simulink model "autosar_swc_actuator"  (R2021a)
settings: Solver=FixedStepDiscrete  StartTime=0.0  StopTime=10.0  FixedStep=0.02  RelTol=1e-3
model workspace (MATLAB code in the model file):
  | HBridgeCmd_LkupTbl = Simulink.LookupTable;
  | HBridgeCmd_LkupTbl.Table.DataType = 'int16';
  | HBridgeCmd_LkupTbl.Table.FieldName = 'Table';
  | HBridgeCmd_LkupTbl.Table.Value = int16( ...
  |   [-2048 -1843 -1638 -1434 -1229 -1024 -819 -614 -410 -205 0 205 410 614 ...
  |    819 1024 1229 1434 1638 1843 2048]);
  | HBridgeCmd_LkupTbl.BreakpointsSpecification = 'Explicit values';
  | HBridgeCmd_LkupTbl.SupportTunableSize = false;
  | HBridgeCmd_LkupTbl.Breakpoints.DataType = 'single';
  | HBridgeCmd_LkupTbl.Breakpoints.FieldName = 'BP1';
  | HBridgeCmd_LkupTbl.Breakpoints.Value = ...
  |   [-100 -90 -80 -70 -60 -50 -40 -30 -20 -10 0 10 20 30 40 50 60 70 80 90 ...
  |    100];
  | HBridgeCmd_LkupTbl.Breakpoints.TunableSizeName = 'N1';
  | HBridgeCmd_LkupTbl.StructTypeInfo.Name = 'MyStruct_Actuator';
  | HBridgeCmd_LkupTbl.StructTypeInfo.HeaderFileName = 'Rte_Type.h';
undefined symbols (not defined in the file): TPSPercentBkpt, TPSPercentTbl
settings Model: Creator=The MathWorks, Inc.  LastModifiedBy=ASUS
settings SolverCC: AlgebraicLoopSolver=TrustRegion
settings DataIOCC: SaveFormat=StructureWithTime  ReturnWorkspaceOutputs=off
settings OptimizationCC: DefaultParameterBehavior=Inlined  PassReuseOutputArgsAs=Individual arguments  ZeroExternalMemoryAtStartup=off  ZeroInternalMemoryAtStartup=off  EfficientTunableParamExpr=on
settings DebuggingCC: ParameterTunabilityLossMsg=error  SFMachineParentedDataDiag=warning  ArithmeticOperatorsInVariantConditions=warning
settings SFSimCC: SimUseLocalCustomCode=off  MATLABDynamicMemAlloc=off  CustomCodeUndefinedFunction=UseInterfaceOnly
settings RTWCC: Description=AUTOSAR  SystemTargetFile=autosar.tlc  GenCodeOnly=on  TemplateMakefile=ert_default_tmf  GenerateReport=on  RTWUseLocalCustomCode=off  IncludeHyperlinkInReport=on  LaunchReport=on  GenerateTraceInfo=on  GenerateTraceReport=on  GenerateTraceReportSl=on  GenerateTraceReportSf=on  GenerateTraceReportEml=on
settings CodeAppCC: ForceParamTrailComments=on  IgnoreCustomStorageClasses=off  OperatorAnnotations=on  SimulinkDataObjDesc=on  SFDataObjDesc=on  InsertBlockDesc=on
settings STFCustomTargetCC: TargetLangStandard=C99 (ISO)  MultiwordLength=256  ParMdlRefBuildCompliant=on  CompOptLevelCompliant=on  IncludeMdlTerminateFcn=off  CombineOutputUpdateFcns=on  SuppressErrorStatus=on  ERTCustomFileBanners=on  SupportNonFinite=off  SupportComplex=off  SupportContinuousTime=off  SupportNonInlinedSFcns=off  RemoveResetFunc=on  MATLABClassNameForMDSCustomization=Simulink.SoftwareTarget.ERTCustomization  CPPClassGenCompliant=on  AutosarCompliant=on  GRTInterface=off  LookupTableObjectStructAxisOrder=2,1,3,4,...  LUTObjectStructOrderEvenSpacing=Size,Table,Breakpoints  SystemTargetFile=autosar.tlc
settings ERTTargetCC: TargetLangStandard=C99 (ISO)  ConcurrentExecutionCompliant=off  IncludeMdlTerminateFcn=off  SuppressErrorStatus=on  SupportNonFinite=off  SupportComplex=off  ModelStepFunctionPrototypeControlCompliant=off  AutosarCompliant=on  LookupTableObjectStructAxisOrder=2,1,3,4,...  LUTObjectStructOrderEvenSpacing=Size,Table,Breakpoints  InlinedParameterPlacement=NonHierarchical  ERTCustomFileTemplate=example_file_process.tlc

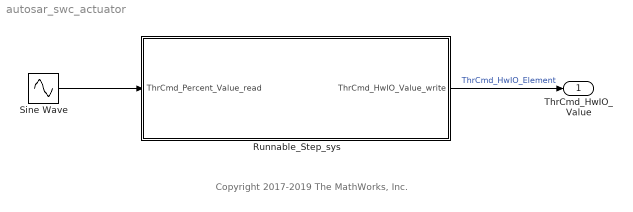
== system autosar_swc_actuator ==
  note: Copyright 2017-2019 The MathWorks, Inc.
  Runnable_Step_sys : Subsystem  TreatAsAtomicUnit=on
  Sine Wave : Sin  Amplitude=100  SampleTime=0
  ThrCmd_HwIO_Value : Outport  OutDataTypeStr=int16  PortDimensions=1  SampleTime=0.02  VectorParamsAs1DForOutWhenUnconnected=off
  wires:
  Runnable_Step_sys/1(ThrCmd_HwIO_Value_write) -> ThrCmd_HwIO_Value/1  "ThrCmd_HwIO_Element"
  Sine Wave/1 -> Runnable_Step_sys/1(ThrCmd_Percent_Value_read)

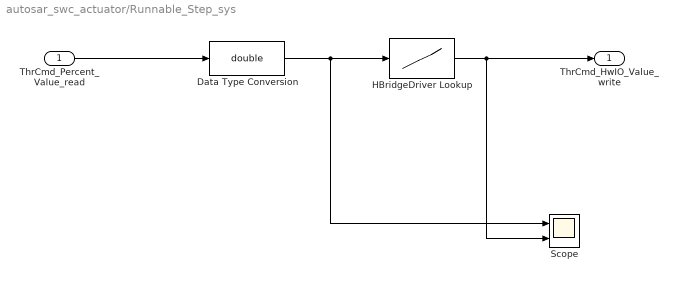
== system autosar_swc_actuator/Runnable_Step_sys ==
  ThrCmd_Percent_Value_read : Inport  SampleTime=0.02
  Data Type Conversion : DataTypeConversion  OutDataTypeStr=double
  HBridgeDriver Lookup : Lookup_n-D  NumberOfTableDimensions=1  DataSpecification=Lookup table object  LookupTableObject=HBridgeCmd_LkupTbl  BreakpointsForDimension1=TPSPercentBkpt  BreakpointsForDimension1DataTypeStr=single  IndexSearchMethod=Linear search  Table=TPSPercentTbl  TableDataTypeStr=single  InterpMethod=Flat  InternalRulePriority=Speed  OutDataTypeStr=Inherit: Inherit from 'Table data'  RndMeth=Simplest  InputSameDT=on
  Scope : Scope  NumInputPorts=2
  ThrCmd_HwIO_Value_write : Outport  SampleTime=0.02  VectorParamsAs1DForOutWhenUnconnected=off
  wires:
  ThrCmd_Percent_Value_read/1 -> Data Type Conversion/1
  HBridgeDriver Lookup/1 -> Scope/2, ThrCmd_HwIO_Value_write/1
  Data Type Conversion/1 -> Scope/1, HBridgeDriver Lookup/1
